simulink library "TM_MASTER"  (Simulink 8.6)
settings: Solver=ode45  StartTime=0.0  StopTime=10.0  RelTol=1e-3
libraries: cdsFilt x75, VIS_LIB x63, cdsEpicsOut x60, cdsTP x48, cdsMuxMatrix x17, cdsFiltCtrl x15, lockin x10, QPD x10, cdsRms x6, FOUROSEM_COILOUTF_MASTER x5, cdsFunctionCall x5, CRYP_TM_MASTER x3
(part 1 of 9)
settings Model: Creator=controls  LastModifiedBy=controls

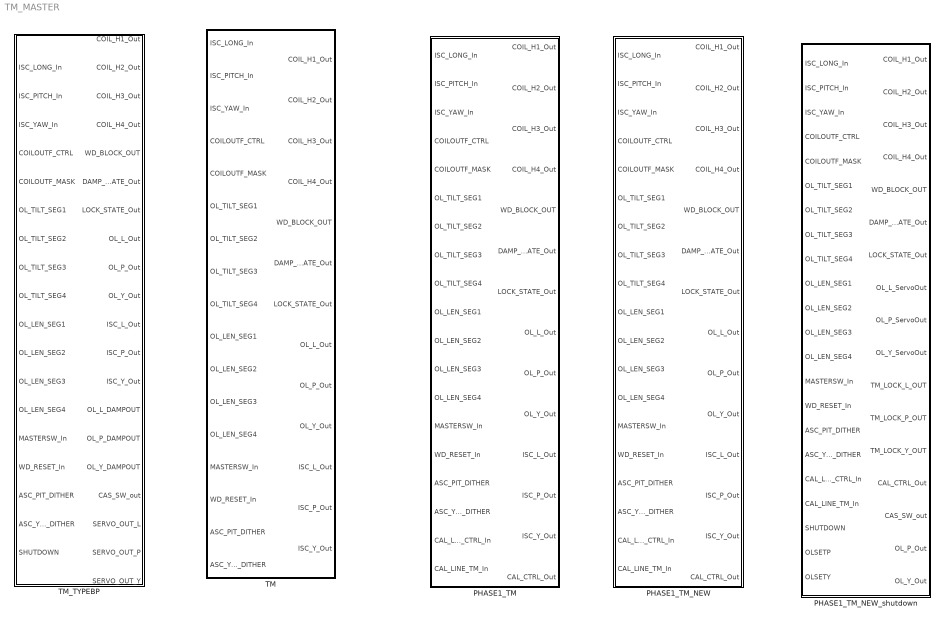
== system TM_MASTER ==
  PHASE1_TM : Subsystem
  PHASE1_TM_NEW : Subsystem
  PHASE1_TM_NEW_shutdown : Subsystem
  TM : Subsystem
  TM_TYPEBP : Subsystem

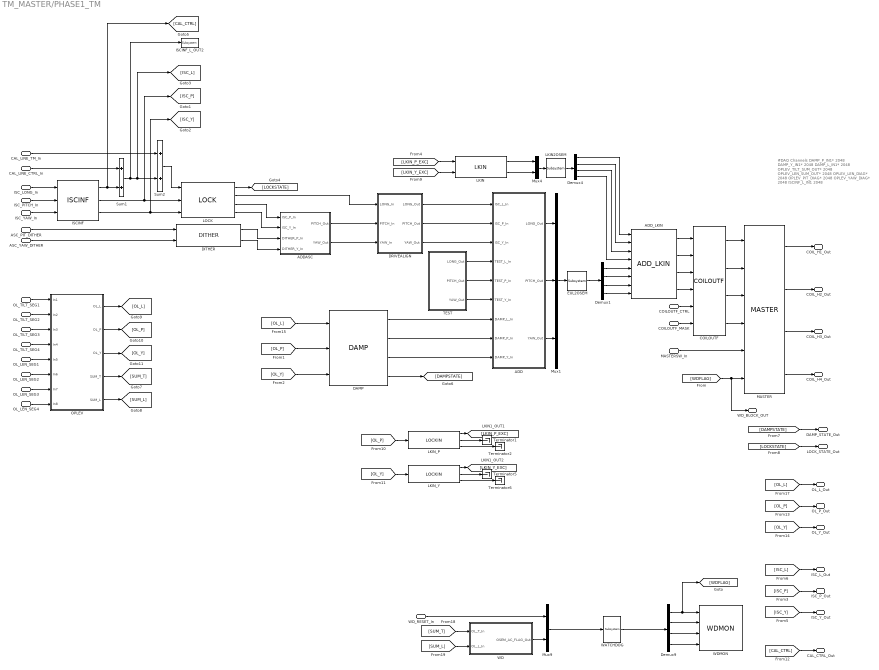
== system TM_MASTER/PHASE1_TM ==
  note: #DAQ Channels
      | DAMP_P_IN1* 2048
      | DAMP_Y_IN1* 2048
      | DAMP_L_IN1* 2048
      | OPLEV_TILT_SUM_OUT* 2048
      | OPLEV_LEN_SUM_OUT* 2048
      | OPLEV_LEN_DIAG* 2048
      | OPLEV_PIT_DIAG* 2048
      | OPLEV_YAW_DIAG* 2048
      | ISCINF_L_IN1 2048
  ISC_LONG_In : Inport
  ISC_PITCH_In : Inport  Port=2
  ISC_YAW_In : Inport  Port=3
  COILOUTF_CTRL : Inport  Port=4
  COILOUTF_MASK : Inport  Port=5
  OL_TILT_SEG1 : Inport  Port=6
  OL_TILT_SEG2 : Inport  Port=7
  OL_TILT_SEG3 : Inport  Port=8
  OL_TILT_SEG4 : Inport  Port=9
  OL_LEN_SEG1 : Inport  Port=10
  OL_LEN_SEG2 : Inport  Port=11
  OL_LEN_SEG3 : Inport  Port=12
  OL_LEN_SEG4 : Inport  Port=13
  MASTERSW_In : Inport  Port=14
  WD_RESET_In : Inport  Port=15
  ASC_PIT_DITHER : Inport  Port=16
  ASC_YAW_DITHER : Inport  Port=17
  CAL_LINE_CTRL_In : Inport  Port=18
  CAL_LINE_TM_In : Inport  Port=19
  ADD : Subsystem
  ADDASC : Subsystem
  ADD_LKIN : VIS_LIB/ADD_LKIN
  COILOUTF : FOUROSEM_COILOUTF_MASTER/COILOUTF
  DAMP : VIS_LIB/DAMP
  DITHER : VIS_LIB/DITHER
  DRIVEALIGN : Subsystem
  Demux1 : Demux
  Demux4 : Demux
  Demux9 : Demux
  EUL2OSEM : cdsMuxMatrix/Subsystem  Tag=cdsMuxMatrix  Description=Any size matrix. Inputs and outputs must be connected using Mux and Demux parts.
      settings: AttributesFormatString=%<Tag>
  ISCINF : VIS_LIB/ISCINF
  ISCINF_L_OUT2 : cdsTP/Subsystem  Tag=Test Point
      settings: AttributesFormatString=%<Tag>
  LKIN : VIS_LIB/LKIN
  LKIN2OSEM : cdsMuxMatrix/Subsystem  Tag=cdsMuxMatrix  Description=Any size matrix. Inputs and outputs must be connected using Mux and Demux parts.
      settings: AttributesFormatString=%<Tag>
  LKIN_P : lockin/LOCKIN  Description=ADL=LOCKIN.adl
      settings: AttributesFormatString=%<Tag>
  LKIN_Y : lockin/LOCKIN  Description=ADL=LOCKIN.adl
      settings: AttributesFormatString=%<Tag>
  LOCK : VIS_LIB/LOCK
  MASTER : CRYP_TM_MASTER/CRYP_TM_MASTER/MASTER
  Mux1 : Mux  Inputs=3
  Mux4 : Mux  Inputs=2
  Mux9 : Mux  Inputs=2
  OPLEV : Subsystem
  Sum1 : Sum
  Sum2 : Sum
  TEST : Subsystem
  Terminator{1..2,5..6} (4 alike) : Terminator
  WATCHDOG : cdsFunctionCall/Subsystem  Tag=cdsFunctionCall  Description=inline OSEMWATCHDOG /opt/rtcds/userapps/release/vis/common/src/WATCHDOG.c
      settings: AttributesFormatString=%<Tag>\n%<Description>
  WD : Subsystem
  WDMON : VIS_LIB/WDMON
  COIL_H1_Out : Outport
  COIL_H2_Out : Outport  Port=2
  COIL_H3_Out : Outport  Port=3
  COIL_H4_Out : Outport  Port=4
  WD_BLOCK_OUT : Outport  Port=5
  DAMP_STATE_Out : Outport  Port=6
  LOCK_STATE_Out : Outport  Port=7
  OL_L_Out : Outport  Port=8
  OL_P_Out : Outport  Port=9
  OL_Y_Out : Outport  Port=10
  ISC_L_Out : Outport  Port=11
  ISC_P_Out : Outport  Port=12
  ISC_Y_Out : Outport  Port=13
  CAL_CTRL_Out : Outport  Port=14
  wires:
  [OL_Y] -> OL_Y_Out/1
  [OL_P] -> OL_P_Out/1
  ISC_PITCH_In/1 -> ISCINF/2
  ISC_LONG_In/1 -> ISCINF/1
  ISC_YAW_In/1 -> ISCINF/3
  WD/1(OSEM_AC_FLAG_Out) -> Mux9/2
  [LKIN_Y_EXC] -> LKIN/2
  [LKIN_P_EXC] -> LKIN/1
  LKIN_Y/3 -> Terminator6/1
  LKIN_Y/2 -> Terminator5/1
  [OL_Y] -> LKIN_Y/1
  LKIN_Y/1 -> [LKIN_Y_EXC]
  LKIN_P/1 -> [LKIN_P_EXC]
  LKIN_P/3 -> Terminator2/1
  LKIN_P/2 -> Terminator1/1
  [OL_P] -> LKIN_P/1
  LOCK/1 -> [LOCKSTATE]
  [LOCKSTATE] -> LOCK_STATE_Out/1
  [DAMPSTATE] -> DAMP_STATE_Out/1
  MASTERSW_In/1 -> MASTER/5
  ADD_LKIN/4 -> COILOUTF/4
  ADD_LKIN/3 -> COILOUTF/3
  ADD_LKIN/2 -> COILOUTF/2
  ADD_LKIN/1 -> COILOUTF/1
  Demux1/4 -> ADD_LKIN/8
  Demux1/3 -> ADD_LKIN/7
  Demux1/2 -> ADD_LKIN/6
  Demux1/1 -> ADD_LKIN/5
  Demux4/4 -> ADD_LKIN/4
  Demux4/3 -> ADD_LKIN/3
  Demux4/2 -> ADD_LKIN/2
  LKIN/2 -> Mux4/2
  LKIN/1 -> Mux4/1
  Demux4/1 -> ADD_LKIN/1
  LKIN2OSEM/1 -> Demux4/1
  Mux4/1 -> LKIN2OSEM/1
  MASTER/4 -> COIL_H4_Out/1
  MASTER/3 -> COIL_H3_Out/1
  MASTER/2 -> COIL_H2_Out/1
  MASTER/1 -> COIL_H1_Out/1
  DRIVEALIGN/3(YAW_Out) -> ADD/3(ISC_Y_In)
  DRIVEALIGN/2(PITCH_Out) -> ADD/2(ISC_P_In)
  DRIVEALIGN/1(LONG_Out) -> ADD/1(ISC_L_In)
  ADDASC/2(YAW_Out) -> DRIVEALIGN/3(YAW_In)
  ADDASC/1(PITCH_Out) -> DRIVEALIGN/2(PITCH_In)
  LOCK/2 -> DRIVEALIGN/1(LONG_In)
  ADD/1(LONG_Out) -> Mux1/1
  ADD/2(PITCH_Out) -> Mux1/2
  ADD/3(YAW_Out) -> Mux1/3
  DITHER/2 -> ADDASC/4(DITHER_Y_In)
  DITHER/1 -> ADDASC/3(DITHER_P_In)
  LOCK/4 -> ADDASC/2(ISC_Y_In)
  ASC_YAW_DITHER/1 -> DITHER/2
  ASC_PIT_DITHER/1 -> DITHER/1
  Mux1/1 -> EUL2OSEM/1
  EUL2OSEM/1 -> Demux1/1
  Demux9/1 -> [WDFLAG], WDMON/1
  Demux9/2 -> WDMON/2
  Demux9/3 -> WDMON/3
  Demux9/4 -> WDMON/4
  WATCHDOG/1 -> Demux9/1
  Mux9/1 -> WATCHDOG/1
  [WDFLAG] -> WD_BLOCK_OUT/1, MASTER/6
  COILOUTF/1 -> MASTER/1
  COILOUTF/2 -> MASTER/2
  COILOUTF/3 -> MASTER/3
  COILOUTF/4 -> MASTER/4
  WD_RESET_In/1 -> Mux9/1
  COILOUTF_MASK/1 -> COILOUTF/6
  COILOUTF_CTRL/1 -> COILOUTF/5
  TEST/1(LONG_Out) -> ADD/4(TEST_L_In)
  TEST/2(PITCH_Out) -> ADD/5(TEST_P_In)
  TEST/3(YAW_Out) -> ADD/6(TEST_Y_In)
  LOCK/3 -> ADDASC/1(ISC_P_In)
  OL_TILT_SEG1/1 -> OPLEV/1(In1)
  OL_TILT_SEG2/1 -> OPLEV/2(In2)
  OL_TILT_SEG4/1 -> OPLEV/4(In4)
  OL_LEN_SEG1/1 -> OPLEV/5(In5)
  OL_LEN_SEG2/1 -> OPLEV/6(In6)
  OL_LEN_SEG3/1 -> OPLEV/7(In7)
  OL_LEN_SEG4/1 -> OPLEV/8(In8)
  OL_TILT_SEG3/1 -> OPLEV/3(In3)
  [OL_L] -> DAMP/1
  DAMP/4 -> [DAMPSTATE]
  DAMP/1 -> ADD/7(DAMP_L_In)
  [SUM_T] -> WD/1(OL_T_In)
  OPLEV/4(SUM_T) -> [SUM_T]
  OPLEV/5(SUM_L) -> [SUM_L]
  [SUM_L] -> WD/2(OL_L_In)
  [OL_L] -> OL_L_Out/1
  OPLEV/1(OL_L) -> [OL_L]
  OPLEV/2(OL_P) -> [OL_P]
  OPLEV/3(OL_Y) -> [OL_Y]
  DAMP/2 -> ADD/8(DAMP_P_In)
  DAMP/3 -> ADD/9(DAMP_Y_In)
  [OL_P] -> DAMP/2
  [OL_Y] -> DAMP/3
  ISCINF/2 -> LOCK/2, [ISC_P]
  ISCINF/3 -> LOCK/3, [ISC_Y]
  [ISC_Y] -> ISC_Y_Out/1
  [ISC_P] -> ISC_P_Out/1
  [ISC_L] -> ISC_L_Out/1
  ISCINF/1 -> [CAL_CTRL], Sum1/2
  CAL_LINE_CTRL_In/1 -> Sum1/1
  Sum1/1 -> ISCINF_L_OUT2/1, [ISC_L], Sum2/2
  CAL_LINE_TM_In/1 -> Sum2/1
  Sum2/1 -> LOCK/1
  [CAL_CTRL] -> CAL_CTRL_Out/1

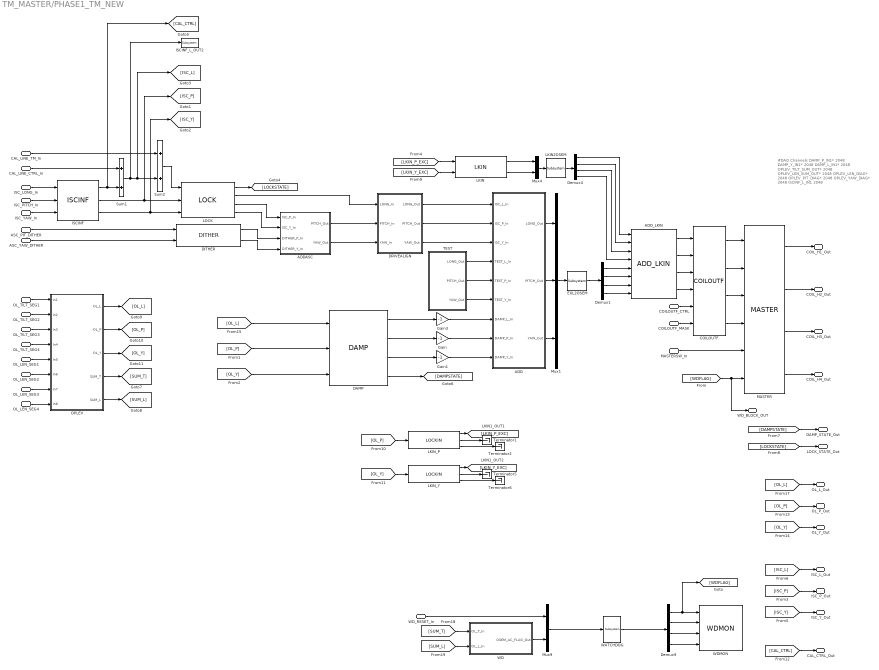
== system TM_MASTER/PHASE1_TM_NEW ==
  note: #DAQ Channels
      | DAMP_P_IN1* 2048
      | DAMP_Y_IN1* 2048
      | DAMP_L_IN1* 2048
      | OPLEV_TILT_SUM_OUT* 2048
      | OPLEV_LEN_SUM_OUT* 2048
      | OPLEV_LEN_DIAG* 2048
      | OPLEV_PIT_DIAG* 2048
      | OPLEV_YAW_DIAG* 2048
      | ISCINF_L_IN1 2048
  ISC_LONG_In : Inport
  ISC_PITCH_In : Inport  Port=2
  ISC_YAW_In : Inport  Port=3
  COILOUTF_CTRL : Inport  Port=4
  COILOUTF_MASK : Inport  Port=5
  OL_TILT_SEG1 : Inport  Port=6
  OL_TILT_SEG2 : Inport  Port=7
  OL_TILT_SEG3 : Inport  Port=8
  OL_TILT_SEG4 : Inport  Port=9
  OL_LEN_SEG1 : Inport  Port=10
  OL_LEN_SEG2 : Inport  Port=11
  OL_LEN_SEG3 : Inport  Port=12
  OL_LEN_SEG4 : Inport  Port=13
  MASTERSW_In : Inport  Port=14
  WD_RESET_In : Inport  Port=15
  ASC_PIT_DITHER : Inport  Port=16
  ASC_YAW_DITHER : Inport  Port=17
  CAL_LINE_CTRL_In : Inport  Port=18
  CAL_LINE_TM_In : Inport  Port=19
  ADD : Subsystem
  ADDASC : Subsystem
  ADD_LKIN : VIS_LIB/ADD_LKIN
  COILOUTF : FOUROSEM_COILOUTF_MASTER/COILOUTF
  DAMP : VIS_LIB/DAMP
  DITHER : VIS_LIB/DITHER
  DRIVEALIGN : Subsystem
  Demux1 : Demux
  Demux4 : Demux
  Demux9 : Demux
  EUL2OSEM : cdsMuxMatrix/Subsystem  Tag=cdsMuxMatrix  Description=Any size matrix. Inputs and outputs must be connected using Mux and Demux parts.
      settings: AttributesFormatString=%<Tag>
  Gain : Gain  Gain=-1
  Gain1 : Gain  Gain=-1
  Gain3 : Gain  Gain=-1
  ISCINF : VIS_LIB/ISCINF
  ISCINF_L_OUT2 : cdsTP/Subsystem  Tag=Test Point
      settings: AttributesFormatString=%<Tag>
  LKIN : VIS_LIB/LKIN
  LKIN2OSEM : cdsMuxMatrix/Subsystem  Tag=cdsMuxMatrix  Description=Any size matrix. Inputs and outputs must be connected using Mux and Demux parts.
      settings: AttributesFormatString=%<Tag>
  LKIN_P : lockin/LOCKIN  Description=ADL=LOCKIN.adl
      settings: AttributesFormatString=%<Tag>
  LKIN_Y : lockin/LOCKIN  Description=ADL=LOCKIN.adl
      settings: AttributesFormatString=%<Tag>
  LOCK : VIS_LIB/LOCK
  MASTER : CRYP_TM_MASTER/CRYP_TM_MASTER/MASTER
  Mux1 : Mux  Inputs=3
  Mux4 : Mux  Inputs=2
  Mux9 : Mux  Inputs=2
  OPLEV : Subsystem
  Sum1 : Sum
  Sum2 : Sum
  TEST : Subsystem
  Terminator{1..2,5..6} (4 alike) : Terminator
  WATCHDOG : cdsFunctionCall/Subsystem  Tag=cdsFunctionCall  Description=inline OSEMWATCHDOG /opt/rtcds/userapps/release/vis/common/src/WATCHDOG.c
      settings: AttributesFormatString=%<Tag>\n%<Description>
  WD : Subsystem
  WDMON : VIS_LIB/WDMON
  COIL_H1_Out : Outport
  COIL_H2_Out : Outport  Port=2
  COIL_H3_Out : Outport  Port=3
  COIL_H4_Out : Outport  Port=4
  WD_BLOCK_OUT : Outport  Port=5
  DAMP_STATE_Out : Outport  Port=6
  LOCK_STATE_Out : Outport  Port=7
  OL_L_Out : Outport  Port=8
  OL_P_Out : Outport  Port=9
  OL_Y_Out : Outport  Port=10
  ISC_L_Out : Outport  Port=11
  ISC_P_Out : Outport  Port=12
  ISC_Y_Out : Outport  Port=13
  CAL_CTRL_Out : Outport  Port=14
  wires:
  [OL_Y] -> OL_Y_Out/1
  [OL_P] -> OL_P_Out/1
  ISC_PITCH_In/1 -> ISCINF/2
  ISC_LONG_In/1 -> ISCINF/1
  ISC_YAW_In/1 -> ISCINF/3
  WD/1(OSEM_AC_FLAG_Out) -> Mux9/2
  [LKIN_Y_EXC] -> LKIN/2
  [LKIN_P_EXC] -> LKIN/1
  LKIN_Y/3 -> Terminator6/1
  LKIN_Y/2 -> Terminator5/1
  [OL_Y] -> LKIN_Y/1
  LKIN_Y/1 -> [LKIN_Y_EXC]
  LKIN_P/1 -> [LKIN_P_EXC]
  LKIN_P/3 -> Terminator2/1
  LKIN_P/2 -> Terminator1/1
  [OL_P] -> LKIN_P/1
  LOCK/1 -> [LOCKSTATE]
  [LOCKSTATE] -> LOCK_STATE_Out/1
  [DAMPSTATE] -> DAMP_STATE_Out/1
  MASTERSW_In/1 -> MASTER/5
  ADD_LKIN/4 -> COILOUTF/4
  ADD_LKIN/3 -> COILOUTF/3
  ADD_LKIN/2 -> COILOUTF/2
  ADD_LKIN/1 -> COILOUTF/1
  Demux1/4 -> ADD_LKIN/8
  Demux1/3 -> ADD_LKIN/7
  Demux1/2 -> ADD_LKIN/6
  Demux1/1 -> ADD_LKIN/5
  Demux4/4 -> ADD_LKIN/4
  Demux4/3 -> ADD_LKIN/3
  Demux4/2 -> ADD_LKIN/2
  LKIN/2 -> Mux4/2
  LKIN/1 -> Mux4/1
  Demux4/1 -> ADD_LKIN/1
  LKIN2OSEM/1 -> Demux4/1
  Mux4/1 -> LKIN2OSEM/1
  MASTER/4 -> COIL_H4_Out/1
  MASTER/3 -> COIL_H3_Out/1
  MASTER/2 -> COIL_H2_Out/1
  MASTER/1 -> COIL_H1_Out/1
  DRIVEALIGN/3(YAW_Out) -> ADD/3(ISC_Y_In)
  DRIVEALIGN/2(PITCH_Out) -> ADD/2(ISC_P_In)
  DRIVEALIGN/1(LONG_Out) -> ADD/1(ISC_L_In)
  ADDASC/2(YAW_Out) -> DRIVEALIGN/3(YAW_In)
  ADDASC/1(PITCH_Out) -> DRIVEALIGN/2(PITCH_In)
  LOCK/2 -> DRIVEALIGN/1(LONG_In)
  ADD/1(LONG_Out) -> Mux1/1
  ADD/2(PITCH_Out) -> Mux1/2
  ADD/3(YAW_Out) -> Mux1/3
  DITHER/2 -> ADDASC/4(DITHER_Y_In)
  DITHER/1 -> ADDASC/3(DITHER_P_In)
  LOCK/4 -> ADDASC/2(ISC_Y_In)
  ASC_YAW_DITHER/1 -> DITHER/2
  ASC_PIT_DITHER/1 -> DITHER/1
  Mux1/1 -> EUL2OSEM/1
  EUL2OSEM/1 -> Demux1/1
  Demux9/1 -> [WDFLAG], WDMON/1
  Demux9/2 -> WDMON/2
  Demux9/3 -> WDMON/3
  Demux9/4 -> WDMON/4
  WATCHDOG/1 -> Demux9/1
  Mux9/1 -> WATCHDOG/1
  [WDFLAG] -> WD_BLOCK_OUT/1, MASTER/6
  COILOUTF/1 -> MASTER/1
  COILOUTF/2 -> MASTER/2
  COILOUTF/3 -> MASTER/3
  COILOUTF/4 -> MASTER/4
  WD_RESET_In/1 -> Mux9/1
  COILOUTF_MASK/1 -> COILOUTF/6
  COILOUTF_CTRL/1 -> COILOUTF/5
  TEST/1(LONG_Out) -> ADD/4(TEST_L_In)
  TEST/2(PITCH_Out) -> ADD/5(TEST_P_In)
  TEST/3(YAW_Out) -> ADD/6(TEST_Y_In)
  LOCK/3 -> ADDASC/1(ISC_P_In)
  OL_TILT_SEG1/1 -> OPLEV/1(In1)
  OL_TILT_SEG2/1 -> OPLEV/2(In2)
  OL_TILT_SEG4/1 -> OPLEV/4(In4)
  OL_LEN_SEG1/1 -> OPLEV/5(In5)
  OL_LEN_SEG2/1 -> OPLEV/6(In6)
  OL_LEN_SEG3/1 -> OPLEV/7(In7)
  OL_LEN_SEG4/1 -> OPLEV/8(In8)
  OL_TILT_SEG3/1 -> OPLEV/3(In3)
  DAMP/4 -> [DAMPSTATE]
  DAMP/1 -> Gain3/1
  [SUM_T] -> WD/1(OL_T_In)
  OPLEV/4(SUM_T) -> [SUM_T]
  OPLEV/5(SUM_L) -> [SUM_L]
  [SUM_L] -> WD/2(OL_L_In)
  [OL_L] -> OL_L_Out/1
  OPLEV/1(OL_L) -> [OL_L]
  OPLEV/2(OL_P) -> [OL_P]
  OPLEV/3(OL_Y) -> [OL_Y]
  DAMP/2 -> Gain/1
  DAMP/3 -> Gain1/1
  ISCINF/2 -> LOCK/2, [ISC_P]
  ISCINF/3 -> LOCK/3, [ISC_Y]
  [ISC_Y] -> ISC_Y_Out/1
  [ISC_P] -> ISC_P_Out/1
  [ISC_L] -> ISC_L_Out/1
  ISCINF/1 -> [CAL_CTRL], Sum1/2
  CAL_LINE_CTRL_In/1 -> Sum1/1
  Sum1/1 -> ISCINF_L_OUT2/1, [ISC_L], Sum2/2
  CAL_LINE_TM_In/1 -> Sum2/1
  Sum2/1 -> LOCK/1
  [CAL_CTRL] -> CAL_CTRL_Out/1
  [OL_L] -> DAMP/1
  [OL_P] -> DAMP/2
  [OL_Y] -> DAMP/3
  Gain3/1 -> ADD/7(DAMP_L_In)
  Gain/1 -> ADD/8(DAMP_P_In)
  Gain1/1 -> ADD/9(DAMP_Y_In)

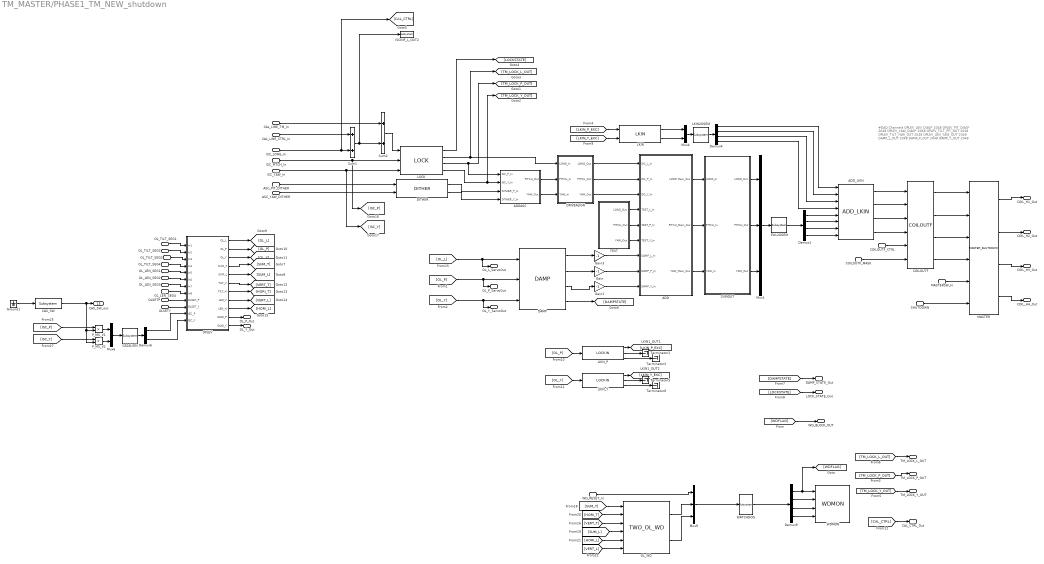
== system TM_MASTER/PHASE1_TM_NEW_shutdown ==
  note: #DAQ Channels
      | OPLEV_LEN_DIAG* 2048
      | OPLEV_PIT_DIAG* 2048
      | OPLEV_YAW_DIAG* 2048
      | OPLEV_TILT_PIT_OUT 2048
      | OPLEV_TILT_YAW_OUT 2048
      | OPLEV_LEN_YAW_OUT 2048
      | DAMP_L_OUT 2048
      | DAMP_P_OUT 2048
      | DAMP_Y_OUT 2048
  ISC_LONG_In : Inport
  ISC_PITCH_In : Inport  Port=2
  ISC_YAW_In : Inport  Port=3
  COILOUTF_CTRL : Inport  Port=4
  COILOUTF_MASK : Inport  Port=5
  OL_TILT_SEG1 : Inport  Port=6
  OL_TILT_SEG2 : Inport  Port=7
  OL_TILT_SEG3 : Inport  Port=8
  OL_TILT_SEG4 : Inport  Port=9
  OL_LEN_SEG1 : Inport  Port=10
  OL_LEN_SEG2 : Inport  Port=11
  OL_LEN_SEG3 : Inport  Port=12
  OL_LEN_SEG4 : Inport  Port=13
  MASTERSW_In : Inport  Port=14
  WD_RESET_In : Inport  Port=15
  ASC_PIT_DITHER : Inport  Port=16
  ASC_YAW_DITHER : Inport  Port=17
  CAL_LINE_CTRL_In : Inport  Port=18
  CAL_LINE_TM_In : Inport  Port=19
  SHUTDOWN : Inport  Port=20
  OLSETP : Inport  Port=21
  OLSETY : Inport  Port=22
  ADD : Subsystem
  ADDASC : Subsystem
  ADD_LKIN : VIS_LIB/ADD_LKIN
  CASALIGN : cdsMuxMatrix/Subsystem  Tag=cdsMuxMatrix  Description=Any size matrix. Inputs and outputs must be connected using Mux and Demux parts.
      settings: AttributesFormatString=%<Tag>
  CAS_SW : cdsEpicsBinIn/Subsystem  Tag=cdsEpicsBinIn  Description=|
      | Purpose:                                                                            
      | Create an EPICS binary (0 or 1) input channel to the FE realtime controls.          
      |                                                                                     
      | Operation:                                                                          
      | Outputs value from an EPICS ai record. Value is binary input (bi Epics record type).
      |                                                                                     
      | Usage:                                                                              
      | Name the part with the desired EPICS channel name.
      settings: AttributesFormatString=%<Tag>
  COILOUTF : FOUROSEM_COILOUTF_MASTER/COILOUTF
  DAMP : VIS_LIB/DAMP
  DITHER : VIS_LIB/DITHER
  DRIVEALIGN : Subsystem
  Demux1 : Demux
  Demux4 : Demux
  Demux6 : Demux  Outputs=2
  Demux9 : Demux
  EUL2OSEM : cdsMuxMatrix/Subsystem  Tag=cdsMuxMatrix  Description=Any size matrix. Inputs and outputs must be connected using Mux and Demux parts.
      settings: AttributesFormatString=%<Tag>
  Gain : Gain  Gain=-1
  Gain1 : Gain  Gain=-1
  Gain3 : Gain  Gain=-1
  Ground1 : Ground
  ISCINF_L_OUT2 : cdsTP/Subsystem  Tag=Test Point
      settings: AttributesFormatString=%<Tag>
  LKIN : VIS_LIB/LKIN
  LKIN2OSEM : cdsMuxMatrix/Subsystem  Tag=cdsMuxMatrix  Description=Any size matrix. Inputs and outputs must be connected using Mux and Demux parts.
      settings: AttributesFormatString=%<Tag>
  LKIN_P : lockin/LOCKIN  Description=ADL=LOCKIN.adl
      settings: AttributesFormatString=%<Tag>
  LKIN_Y : lockin/LOCKIN  Description=ADL=LOCKIN.adl
      settings: AttributesFormatString=%<Tag>
  LOCK : VIS_LIB/LOCK
  MASTER : VIS_LIB/MASTER_SHUTDOWN
  Mux1 : Mux  Inputs=3
  Mux4 : Mux  Inputs=2
  Mux6 : Mux  Inputs=2
  Mux9 : Mux  Inputs=3
  OL_WD : OPLEV_MASTER/TWO_OL_WD
  OPLEV : Subsystem
  P_MS_V1 : Product  RndMeth=Zero
  P_MS_V2 : Product  RndMeth=Zero
  SUMOUT : Subsystem
  Sum1 : Sum
  Sum2 : Sum
  TEST : Subsystem
  Terminator{1..2,5..6} (4 alike) : Terminator
  WATCHDOG : cdsFunctionCall/Subsystem  Tag=cdsFunctionCall  Description=inline OPLEVWATCHDOG /opt/rtcds/userapps/release/vis/common/src/WATCHDOG.c
      settings: AttributesFormatString=%<Tag>\n%<Description>
  WDMON : VIS_LIB/WDMON
  COIL_H1_Out : Outport
  COIL_H2_Out : Outport  Port=2
  COIL_H3_Out : Outport  Port=3
  COIL_H4_Out : Outport  Port=4
  WD_BLOCK_OUT : Outport  Port=5
  DAMP_STATE_Out : Outport  Port=6
  LOCK_STATE_Out : Outport  Port=7
  OL_L_ServoOut : Outport  Port=8
  OL_P_ServoOut : Outport  Port=9
  OL_Y_ServoOut : Outport  Port=10
  TM_LOCK_L_OUT : Outport  Port=11
  TM_LOCK_P_OUT : Outport  Port=12
  TM_LOCK_Y_OUT : Outport  Port=13
  CAL_CTRL_Out : Outport  Port=14
  CAS_SW_out : Outport  Port=15
  OL_P_Out : Outport  Port=16
  OL_Y_Out : Outport  Port=17
  wires:
  CASALIGN/1 -> Demux6/1
  Mux6/1 -> CASALIGN/1
  P_MS_V2/1 -> Mux6/2
  P_MS_V1/1 -> Mux6/1
  CAS_SW/1 -> CAS_SW_out/1, P_MS_V2/2, P_MS_V1/2
  [ISC_P] -> P_MS_V1/1
  [ISC_Y] -> P_MS_V2/1
  Ground1/1 -> CAS_SW/1
  OPLEV/3(OL_Y) -> [OL_Y]
  SUMOUT/3(YAW_Out) -> Mux1/3
  SUMOUT/2(PITCH_Out) -> Mux1/2
  SUMOUT/1(LONG_Out) -> Mux1/1
  OL_WD/1 -> Mux9/2
  [LKIN_Y_EXC] -> LKIN/2
  [LKIN_P_EXC] -> LKIN/1
  LKIN_Y/3 -> Terminator6/1
  LKIN_Y/2 -> Terminator5/1
  [OL_Y] -> LKIN_Y/1
  LKIN_Y/1 -> [LKIN_Y_EXC]
  LKIN_P/1 -> [LKIN_P_EXC]
  LKIN_P/3 -> Terminator2/1
  LKIN_P/2 -> Terminator1/1
  [OL_P] -> LKIN_P/1
  LOCK/1 -> [LOCKSTATE]
  [LOCKSTATE] -> LOCK_STATE_Out/1
  [DAMPSTATE] -> DAMP_STATE_Out/1
  MASTERSW_In/1 -> MASTER/5
  ADD_LKIN/4 -> COILOUTF/4
  ADD_LKIN/3 -> COILOUTF/3
  ADD_LKIN/2 -> COILOUTF/2
  ADD_LKIN/1 -> COILOUTF/1
  Demux1/4 -> ADD_LKIN/8
  Demux1/3 -> ADD_LKIN/7
  Demux1/2 -> ADD_LKIN/6
  Demux1/1 -> ADD_LKIN/5
  Demux4/4 -> ADD_LKIN/4
  Demux4/3 -> ADD_LKIN/3
  Demux4/2 -> ADD_LKIN/2
  LKIN/2 -> Mux4/2
  LKIN/1 -> Mux4/1
  Demux4/1 -> ADD_LKIN/1
  LKIN2OSEM/1 -> Demux4/1
  Mux4/1 -> LKIN2OSEM/1
  MASTER/4 -> COIL_H4_Out/1
  MASTER/3 -> COIL_H3_Out/1
  MASTER/2 -> COIL_H2_Out/1
  MASTER/1 -> COIL_H1_Out/1
  DRIVEALIGN/3(YAW_Out) -> ADD/3(ISC_Y_In)
  DRIVEALIGN/2(PITCH_Out) -> ADD/2(ISC_P_In)
  DRIVEALIGN/1(LONG_Out) -> ADD/1(ISC_L_In)
  ADDASC/2(YAW_Out) -> DRIVEALIGN/3(YAW_In)
  ADDASC/1(PITCH_Out) -> DRIVEALIGN/2(PITCH_In)
  LOCK/2 -> [TM_LOCK_L_OUT], DRIVEALIGN/1(LONG_In)
  ADD/1(LONG Main_Out) -> SUMOUT/1(LONG_In)
  ADD/2(PITCH_Main_Out) -> SUMOUT/2(PITCH_In)
  ADD/3(YAW_Main_Out) -> SUMOUT/3(YAW_In)
  DITHER/2 -> ADDASC/4(DITHER_Y_In)
  DITHER/1 -> ADDASC/3(DITHER_P_In)
  LOCK/4 -> [TM_LOCK_Y_OUT], ADDASC/2(ISC_Y_In)
  ASC_YAW_DITHER/1 -> DITHER/2
  ASC_PIT_DITHER/1 -> DITHER/1
  Mux1/1 -> EUL2OSEM/1
  EUL2OSEM/1 -> Demux1/1
  Demux9/1 -> [WDFLAG], WDMON/1
  Demux9/2 -> WDMON/2
  Demux9/3 -> WDMON/3
  Demux9/4 -> WDMON/4
  WATCHDOG/1 -> Demux9/1
  Mux9/1 -> WATCHDOG/1
  [WDFLAG] -> WD_BLOCK_OUT/1
  COILOUTF/1 -> MASTER/1
  COILOUTF/2 -> MASTER/2
  COILOUTF/3 -> MASTER/3
  COILOUTF/4 -> MASTER/4
  WD_RESET_In/1 -> Mux9/1
  COILOUTF_MASK/1 -> COILOUTF/6
  COILOUTF_CTRL/1 -> COILOUTF/5
  TEST/1(LONG_Out) -> ADD/4(TEST_L_In)
  TEST/2(PITCH_Out) -> ADD/5(TEST_P_In)
  TEST/3(YAW_Out) -> ADD/6(TEST_Y_In)
  LOCK/3 -> [TM_LOCK_P_OUT], ADDASC/1(ISC_P_In)
  OL_TILT_SEG1/1 -> OPLEV/1(In1)
  OL_TILT_SEG2/1 -> OPLEV/2(In2)
  OL_TILT_SEG4/1 -> OPLEV/4(In4)
  OL_LEN_SEG1/1 -> OPLEV/5(In5)
  OL_LEN_SEG2/1 -> OPLEV/6(In6)
  OL_LEN_SEG3/1 -> OPLEV/7(In7)
  OL_LEN_SEG4/1 -> OPLEV/8(In8)
  OL_TILT_SEG3/1 -> OPLEV/3(In3)
  DAMP/4 -> [DAMPSTATE]
  DAMP/1 -> Gain3/1
  [SUM_T] -> OL_WD/1
  OPLEV/4(SUM_T) -> [SUM_T]
  OPLEV/5(SUM_L) -> [SUM_L]
  [SUM_L] -> OL_WD/4
  OPLEV/1(OL_L) -> [OL_L]
  DAMP/2 -> Gain/1
  DAMP/3 -> Gain1/1
  ISC_PITCH_In/1 -> LOCK/2, [ISC_P]
  ISC_YAW_In/1 -> LOCK/3, [ISC_Y]
  [TM_LOCK_Y_OUT] -> TM_LOCK_Y_OUT/1
  [TM_LOCK_P_OUT] -> TM_LOCK_P_OUT/1
  [TM_LOCK_L_OUT] -> TM_LOCK_L_OUT/1
  ISC_LONG_In/1 -> [CAL_CTRL], Sum1/2
  CAL_LINE_CTRL_In/1 -> Sum1/1
  Sum1/1 -> ISCINF_L_OUT2/1, Sum2/2
  CAL_LINE_TM_In/1 -> Sum2/1
  Sum2/1 -> LOCK/1
  [CAL_CTRL] -> CAL_CTRL_Out/1
  [OL_L] -> OL_L_ServoOut/1, DAMP/1
  SHUTDOWN/1 -> MASTER/6
  OPLEV/6(TILT_V) -> [VERT_T]
  OPLEV/7(TILT_H) -> [HORI_T]
  OPLEV/8(LEN_V) -> [VERT_L]
  OPLEV/9(LEN_H) -> [HORI_L]
  OL_WD/2 -> Mux9/3
  [VERT_T] -> OL_WD/3
  [HORI_T] -> OL_WD/2
  [HORI_L] -> OL_WD/5
  [VERT_L] -> OL_WD/6
  OPLEV/2(OL_P) -> [OL_P]
  Demux6/1 -> OPLEV/11(ISC_P)
  Demux6/2 -> OPLEV/12(ISC_Y)
  Gain3/1 -> ADD/7(DAMP_L_In)
  Gain/1 -> ADD/8(DAMP_P_In)
  Gain1/1 -> ADD/9(DAMP_Y_In)
  [OL_P] -> OL_P_ServoOut/1, DAMP/2
  [OL_Y] -> OL_Y_ServoOut/1, DAMP/3
  OLSETP/1 -> OPLEV/9(OLSET_P)
  OLSETY/1 -> OPLEV/10(OLSET_Y)
  OPLEV/10(DIAG_P) -> OL_P_Out/1
  OPLEV/11(DIAG_Y) -> OL_Y_Out/1

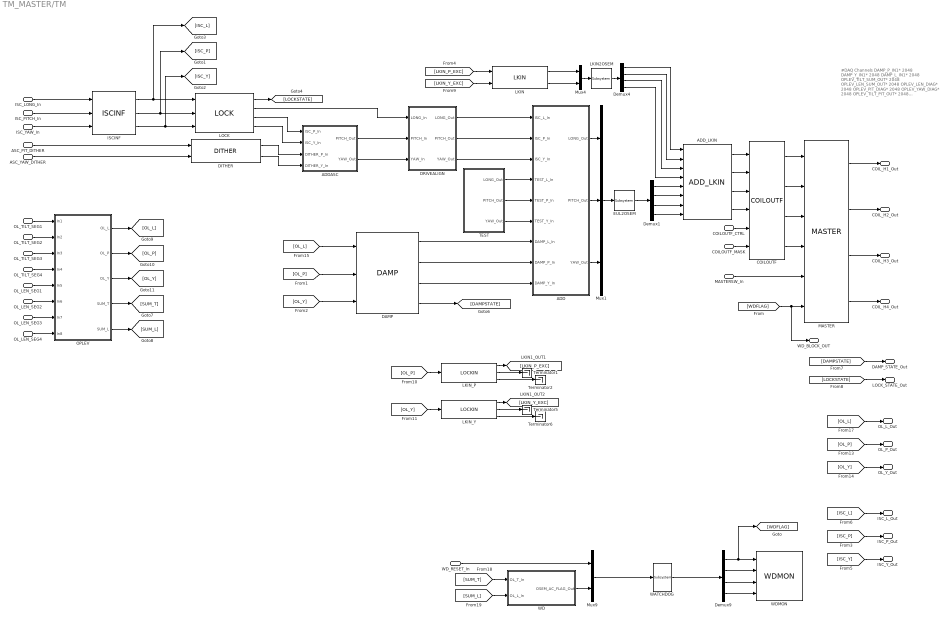
== system TM_MASTER/TM ==
  note: #DAQ Channels
      | DAMP_P_IN1* 2048
      | DAMP_Y_IN1* 2048
      | DAMP_L_IN1* 2048
      | OPLEV_TILT_SUM_OUT* 2048
      | OPLEV_LEN_SUM_OUT* 2048
      | OPLEV_LEN_DIAG* 2048
      | OPLEV_PIT_DIAG* 2048
      | OPLEV_YAW_DIAG* 2048
      | OPLEV_TILT_PIT_OUT* 2048
      | OPLEV_TILT_YAW_OUT* 2048
      | ISCINF_L_IN1 2048
  ISC_LONG_In : Inport
  ISC_PITCH_In : Inport  Port=2
  ISC_YAW_In : Inport  Port=3
  COILOUTF_CTRL : Inport  Port=4
  COILOUTF_MASK : Inport  Port=5
  OL_TILT_SEG1 : Inport  Port=6
  OL_TILT_SEG2 : Inport  Port=7
  OL_TILT_SEG3 : Inport  Port=8
  OL_TILT_SEG4 : Inport  Port=9
  OL_LEN_SEG1 : Inport  Port=10
  OL_LEN_SEG2 : Inport  Port=11
  OL_LEN_SEG3 : Inport  Port=12
  OL_LEN_SEG4 : Inport  Port=13
  MASTERSW_In : Inport  Port=14
  WD_RESET_In : Inport  Port=15
  ASC_PIT_DITHER : Inport  Port=16
  ASC_YAW_DITHER : Inport  Port=17
  ADD : Subsystem
  ADDASC : Subsystem
  ADD_LKIN : VIS_LIB/ADD_LKIN
  COILOUTF : FOUROSEM_COILOUTF_MASTER/COILOUTF
  DAMP : VIS_LIB/DAMP
  DITHER : VIS_LIB/DITHER
  DRIVEALIGN : Subsystem
  Demux1 : Demux
  Demux4 : Demux
  Demux9 : Demux
  EUL2OSEM : cdsMuxMatrix/Subsystem  Tag=cdsMuxMatrix  Description=Any size matrix. Inputs and outputs must be connected using Mux and Demux parts.
      settings: AttributesFormatString=%<Tag>
  ISCINF : VIS_LIB/ISCINF
  LKIN : VIS_LIB/LKIN
  LKIN2OSEM : cdsMuxMatrix/Subsystem  Tag=cdsMuxMatrix  Description=Any size matrix. Inputs and outputs must be connected using Mux and Demux parts.
      settings: AttributesFormatString=%<Tag>
  LKIN_P : lockin/LOCKIN  Description=ADL=LOCKIN.adl
      settings: AttributesFormatString=%<Tag>
  LKIN_Y : lockin/LOCKIN  Description=ADL=LOCKIN.adl
      settings: AttributesFormatString=%<Tag>
  LOCK : VIS_LIB/LOCK
  MASTER : CRYP_TM_MASTER/CRYP_TM_MASTER/MASTER
  Mux1 : Mux  Inputs=3
  Mux4 : Mux  Inputs=2
  Mux9 : Mux  Inputs=2
  OPLEV : Subsystem
  TEST : Subsystem
  Terminator{1..2,5..6} (4 alike) : Terminator
  WATCHDOG : cdsFunctionCall/Subsystem  Tag=cdsFunctionCall  Description=inline OSEMWATCHDOG /opt/rtcds/userapps/release/vis/common/src/WATCHDOG.c
      settings: AttributesFormatString=%<Tag>\n%<Description>
  WD : Subsystem
  WDMON : VIS_LIB/WDMON
  COIL_H1_Out : Outport
  COIL_H2_Out : Outport  Port=2
  COIL_H3_Out : Outport  Port=3
  COIL_H4_Out : Outport  Port=4
  WD_BLOCK_OUT : Outport  Port=5
  DAMP_STATE_Out : Outport  Port=6
  LOCK_STATE_Out : Outport  Port=7
  OL_L_Out : Outport  Port=8
  OL_P_Out : Outport  Port=9
  OL_Y_Out : Outport  Port=10
  ISC_L_Out : Outport  Port=11
  ISC_P_Out : Outport  Port=12
  ISC_Y_Out : Outport  Port=13
  wires:
  [OL_Y] -> OL_Y_Out/1
  [OL_P] -> OL_P_Out/1
  ISC_PITCH_In/1 -> ISCINF/2
  ISC_LONG_In/1 -> ISCINF/1
  ISC_YAW_In/1 -> ISCINF/3
  WD/1(OSEM_AC_FLAG_Out) -> Mux9/2
  [LKIN_Y_EXC] -> LKIN/2
  [LKIN_P_EXC] -> LKIN/1
  LKIN_Y/3 -> Terminator6/1
  LKIN_Y/2 -> Terminator5/1
  [OL_Y] -> LKIN_Y/1
  LKIN_Y/1 -> [LKIN_Y_EXC]
  LKIN_P/1 -> [LKIN_P_EXC]
  LKIN_P/3 -> Terminator2/1
  LKIN_P/2 -> Terminator1/1
  [OL_P] -> LKIN_P/1
  LOCK/1 -> [LOCKSTATE]
  [LOCKSTATE] -> LOCK_STATE_Out/1
  [DAMPSTATE] -> DAMP_STATE_Out/1
  MASTERSW_In/1 -> MASTER/5
  ADD_LKIN/4 -> COILOUTF/4
  ADD_LKIN/3 -> COILOUTF/3
  ADD_LKIN/2 -> COILOUTF/2
  ADD_LKIN/1 -> COILOUTF/1
  Demux1/4 -> ADD_LKIN/8
  Demux1/3 -> ADD_LKIN/7
  Demux1/2 -> ADD_LKIN/6
  Demux1/1 -> ADD_LKIN/5
  Demux4/4 -> ADD_LKIN/4
  Demux4/3 -> ADD_LKIN/3
  Demux4/2 -> ADD_LKIN/2
  LKIN/2 -> Mux4/2
  LKIN/1 -> Mux4/1
  Demux4/1 -> ADD_LKIN/1
  LKIN2OSEM/1 -> Demux4/1
  Mux4/1 -> LKIN2OSEM/1
  MASTER/4 -> COIL_H4_Out/1
  MASTER/3 -> COIL_H3_Out/1
  MASTER/2 -> COIL_H2_Out/1
  MASTER/1 -> COIL_H1_Out/1
  DRIVEALIGN/3(YAW_Out) -> ADD/3(ISC_Y_In)
  DRIVEALIGN/2(PITCH_Out) -> ADD/2(ISC_P_In)
  DRIVEALIGN/1(LONG_Out) -> ADD/1(ISC_L_In)
  ADDASC/2(YAW_Out) -> DRIVEALIGN/3(YAW_In)
  ADDASC/1(PITCH_Out) -> DRIVEALIGN/2(PITCH_In)
  LOCK/2 -> DRIVEALIGN/1(LONG_In)
  ADD/1(LONG_Out) -> Mux1/1
  ADD/2(PITCH_Out) -> Mux1/2
  ADD/3(YAW_Out) -> Mux1/3
  DITHER/2 -> ADDASC/4(DITHER_Y_In)
  DITHER/1 -> ADDASC/3(DITHER_P_In)
  LOCK/4 -> ADDASC/2(ISC_Y_In)
  ASC_YAW_DITHER/1 -> DITHER/2
  ASC_PIT_DITHER/1 -> DITHER/1
  Mux1/1 -> EUL2OSEM/1
  EUL2OSEM/1 -> Demux1/1
  Demux9/1 -> [WDFLAG], WDMON/1
  Demux9/2 -> WDMON/2
  Demux9/3 -> WDMON/3
  Demux9/4 -> WDMON/4
  WATCHDOG/1 -> Demux9/1
  Mux9/1 -> WATCHDOG/1
  [WDFLAG] -> WD_BLOCK_OUT/1, MASTER/6
  COILOUTF/1 -> MASTER/1
  COILOUTF/2 -> MASTER/2
  COILOUTF/3 -> MASTER/3
  COILOUTF/4 -> MASTER/4
  WD_RESET_In/1 -> Mux9/1
  COILOUTF_MASK/1 -> COILOUTF/6
  COILOUTF_CTRL/1 -> COILOUTF/5
  TEST/1(LONG_Out) -> ADD/4(TEST_L_In)
  TEST/2(PITCH_Out) -> ADD/5(TEST_P_In)
  TEST/3(YAW_Out) -> ADD/6(TEST_Y_In)
  LOCK/3 -> ADDASC/1(ISC_P_In)
  OL_TILT_SEG1/1 -> OPLEV/1(In1)
  OL_TILT_SEG2/1 -> OPLEV/2(In2)
  OL_TILT_SEG4/1 -> OPLEV/4(In4)
  OL_LEN_SEG1/1 -> OPLEV/5(In5)
  OL_LEN_SEG2/1 -> OPLEV/6(In6)
  OL_LEN_SEG3/1 -> OPLEV/7(In7)
  OL_LEN_SEG4/1 -> OPLEV/8(In8)
  OL_TILT_SEG3/1 -> OPLEV/3(In3)
  [OL_L] -> DAMP/1
  DAMP/4 -> [DAMPSTATE]
  DAMP/1 -> ADD/7(DAMP_L_In)
  [SUM_T] -> WD/1(OL_T_In)
  OPLEV/4(SUM_T) -> [SUM_T]
  OPLEV/5(SUM_L) -> [SUM_L]
  [SUM_L] -> WD/2(OL_L_In)
  [OL_L] -> OL_L_Out/1
  OPLEV/1(OL_L) -> [OL_L]
  OPLEV/2(OL_P) -> [OL_P]
  OPLEV/3(OL_Y) -> [OL_Y]
  DAMP/2 -> ADD/8(DAMP_P_In)
  DAMP/3 -> ADD/9(DAMP_Y_In)
  [OL_P] -> DAMP/2
  [OL_Y] -> DAMP/3
  ISCINF/1 -> [ISC_L], LOCK/1
  ISCINF/2 -> [ISC_P], LOCK/2
  ISCINF/3 -> [ISC_Y], LOCK/3
  [ISC_Y] -> ISC_Y_Out/1
  [ISC_P] -> ISC_P_Out/1
  [ISC_L] -> ISC_L_Out/1

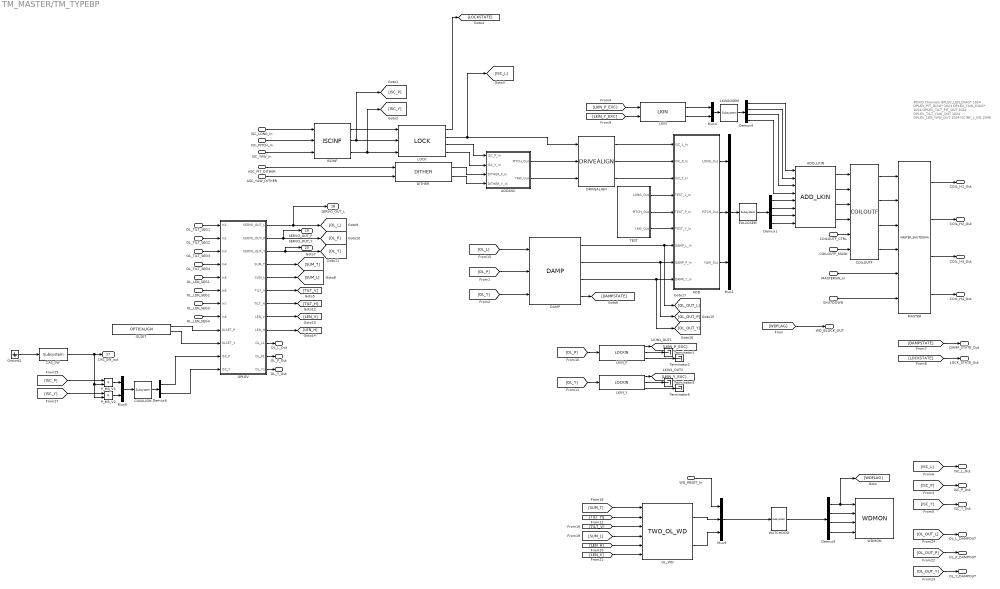
== system TM_MASTER/TM_TYPEBP ==
  note: #DAQ Channels
      | OPLEV_LEN_DIAG* 1024
      | OPLEV_PIT_DIAG* 1024
      | OPLEV_YAW_DIAG* 1024
      | OPLEV_TILT_PIT_OUT 1024
      | OPLEV_TILT_YAW_OUT 1024
      | OPLEV_LEN_YAW_OUT 1024
      | ISCINF_L_IN1 2048
  ISC_LONG_In : Inport
  ISC_PITCH_In : Inport  Port=2
  ISC_YAW_In : Inport  Port=3
  COILOUTF_CTRL : Inport  Port=4
  COILOUTF_MASK : Inport  Port=5
  OL_TILT_SEG1 : Inport  Port=6
  OL_TILT_SEG2 : Inport  Port=7
  OL_TILT_SEG3 : Inport  Port=8
  OL_TILT_SEG4 : Inport  Port=9
  OL_LEN_SEG1 : Inport  Port=10
  OL_LEN_SEG2 : Inport  Port=11
  OL_LEN_SEG3 : Inport  Port=12
  OL_LEN_SEG4 : Inport  Port=13
  MASTERSW_In : Inport  Port=14
  WD_RESET_In : Inport  Port=15
  ASC_PIT_DITHER : Inport  Port=16
  ASC_YAW_DITHER : Inport  Port=17
  SHUTDOWN : Inport  Port=18
  ADD : Subsystem
  ADDASC : Subsystem
  ADD_LKIN : VIS_LIB/ADD_LKIN
  CASALIGN : cdsMuxMatrix/Subsystem  Tag=cdsMuxMatrix  Description=Any size matrix. Inputs and outputs must be connected using Mux and Demux parts.
      settings: AttributesFormatString=%<Tag>
  CAS_SW : cdsEpicsBinIn/Subsystem  Tag=cdsEpicsBinIn  Description=|
      | Purpose:                                                                            
      | Create an EPICS binary (0 or 1) input channel to the FE realtime controls.          
      |                                                                                     
      | Operation:                                                                          
      | Outputs value from an EPICS ai record. Value is binary input (bi Epics record type).
      |                                                                                     
      | Usage:                                                                              
      | Name the part with the desired EPICS channel name.
      settings: AttributesFormatString=%<Tag>
  COILOUTF : FOUROSEM_COILOUTF_MASTER/COILOUTF
  DAMP : VIS_LIB/DAMP
  DITHER : VIS_LIB/DITHER
  DRIVEALIGN : VIS_LIB/DRIVEALIGN
  Demux1 : Demux
  Demux4 : Demux
  Demux6 : Demux  Outputs=2
  Demux9 : Demux
  EUL2OSEM : cdsMuxMatrix/Subsystem  Tag=cdsMuxMatrix  Description=Any size matrix. Inputs and outputs must be connected using Mux and Demux parts.
      settings: AttributesFormatString=%<Tag>
  Ground1 : Ground
  ISCINF : VIS_LIB/ISCINF
  LKIN : VIS_LIB/LKIN
  LKIN2OSEM : cdsMuxMatrix/Subsystem  Tag=cdsMuxMatrix  Description=Any size matrix. Inputs and outputs must be connected using Mux and Demux parts.
      settings: AttributesFormatString=%<Tag>
  LKIN_P : lockin/LOCKIN  Description=ADL=LOCKIN.adl
      settings: AttributesFormatString=%<Tag>
  LKIN_Y : lockin/LOCKIN  Description=ADL=LOCKIN.adl
      settings: AttributesFormatString=%<Tag>
  LOCK : VIS_LIB/LOCK
  MASTER : VIS_LIB/MASTER_SHUTDOWN
  Mux1 : Mux  Inputs=3
  Mux4 : Mux  Inputs=2
  Mux6 : Mux  Inputs=2
  Mux9 : Mux  Inputs=3
  OLSET : SIXOSEM_F_STAGE_MASTER/SIXOSEM_F_STAGE_TYPEBP_MASTER/OPTICALIGN
  OL_WD : OPLEV_MASTER/TWO_OL_WD
  OPLEV : Subsystem
  P_MS_V1 : Product  RndMeth=Zero
  P_MS_V2 : Product  RndMeth=Zero
  TEST : Subsystem
  Terminator{1..2,5..6} (4 alike) : Terminator
  WATCHDOG : cdsFunctionCall/Subsystem  Tag=cdsFunctionCall  Description=inline OPLEVWATCHDOG /opt/rtcds/userapps/release/vis/common/src/WATCHDOG.c
      settings: AttributesFormatString=%<Tag>\n%<Description>
  WDMON : VIS_LIB/WDMON
  COIL_H1_Out : Outport
  COIL_H2_Out : Outport  Port=2
  COIL_H3_Out : Outport  Port=3
  COIL_H4_Out : Outport  Port=4
  WD_BLOCK_OUT : Outport  Port=5
  DAMP_STATE_Out : Outport  Port=6
  LOCK_STATE_Out : Outport  Port=7
  OL_L_Out : Outport  Port=8
  OL_P_Out : Outport  Port=9
  OL_Y_Out : Outport  Port=10
  ISC_L_Out : Outport  Port=11
  ISC_P_Out : Outport  Port=12
  ISC_Y_Out : Outport  Port=13
  OL_L_DAMPOUT : Outport  Port=14
  OL_P_DAMPOUT : Outport  Port=15
  OL_Y_DAMPOUT : Outport  Port=16
  CAS_SW_out : Outport  Port=17
  SERVO_OUT_L : Outport  Port=18
  SERVO_OUT_P : Outport  Port=19
  SERVO_OUT_Y : Outport  Port=20
  wires:
  ISC_PITCH_In/1 -> ISCINF/2
  ISC_LONG_In/1 -> ISCINF/1
  ISC_YAW_In/1 -> ISCINF/3
  OL_WD/1 -> Mux9/2
  [LKIN_Y_EXC] -> LKIN/2
  [LKIN_P_EXC] -> LKIN/1
  LKIN_Y/3 -> Terminator6/1
  LKIN_Y/2 -> Terminator5/1
  [OL_Y] -> LKIN_Y/1
  LKIN_Y/1 -> [LKIN_Y_EXC]
  LKIN_P/1 -> [LKIN_P_EXC]
  LKIN_P/3 -> Terminator2/1
  LKIN_P/2 -> Terminator1/1
  [OL_P] -> LKIN_P/1
  LOCK/1 -> [LOCKSTATE]
  [LOCKSTATE] -> LOCK_STATE_Out/1
  [DAMPSTATE] -> DAMP_STATE_Out/1
  MASTERSW_In/1 -> MASTER/5
  ADD_LKIN/4 -> COILOUTF/4
  ADD_LKIN/3 -> COILOUTF/3
  ADD_LKIN/2 -> COILOUTF/2
  ADD_LKIN/1 -> COILOUTF/1
  Demux1/4 -> ADD_LKIN/8
  Demux1/3 -> ADD_LKIN/7
  Demux1/2 -> ADD_LKIN/6
  Demux1/1 -> ADD_LKIN/5
  Demux4/4 -> ADD_LKIN/4
  Demux4/3 -> ADD_LKIN/3
  Demux4/2 -> ADD_LKIN/2
  LKIN/2 -> Mux4/2
  LKIN/1 -> Mux4/1
  Demux4/1 -> ADD_LKIN/1
  LKIN2OSEM/1 -> Demux4/1
  Mux4/1 -> LKIN2OSEM/1
  MASTER/4 -> COIL_H4_Out/1
  MASTER/3 -> COIL_H3_Out/1
  MASTER/2 -> COIL_H2_Out/1
  MASTER/1 -> COIL_H1_Out/1
  DRIVEALIGN/3 -> ADD/3(ISC_Y_In)
  DRIVEALIGN/2 -> ADD/2(ISC_P_In)
  DRIVEALIGN/1 -> ADD/1(ISC_L_In)
  ADDASC/2(YAW_Out) -> DRIVEALIGN/3
  ADDASC/1(PITCH_Out) -> DRIVEALIGN/2
  LOCK/2 -> [ISC_L], DRIVEALIGN/1
  ADD/1(LONG_Out) -> Mux1/1
  ADD/2(PITCH_Out) -> Mux1/2
  ADD/3(YAW_Out) -> Mux1/3
  DITHER/2 -> ADDASC/4(DITHER_Y_In)
  DITHER/1 -> ADDASC/3(DITHER_P_In)
  LOCK/4 -> ADDASC/2(ISC_Y_In)
  ASC_YAW_DITHER/1 -> DITHER/2
  ASC_PIT_DITHER/1 -> DITHER/1
  Mux1/1 -> EUL2OSEM/1
  EUL2OSEM/1 -> Demux1/1
  Demux9/1 -> [WDFLAG], WDMON/1
  Demux9/2 -> WDMON/2
  Demux9/3 -> WDMON/3
  Demux9/4 -> WDMON/4
  WATCHDOG/1 -> Demux9/1
  Mux9/1 -> WATCHDOG/1
  [WDFLAG] -> WD_BLOCK_OUT/1
  COILOUTF/1 -> MASTER/1
  COILOUTF/2 -> MASTER/2
  COILOUTF/3 -> MASTER/3
  COILOUTF/4 -> MASTER/4
  WD_RESET_In/1 -> Mux9/1
  COILOUTF_MASK/1 -> COILOUTF/6
  COILOUTF_CTRL/1 -> COILOUTF/5
  TEST/1(LONG_Out) -> ADD/4(TEST_L_In)
  TEST/2(PITCH_Out) -> ADD/5(TEST_P_In)
  TEST/3(YAW_Out) -> ADD/6(TEST_Y_In)
  LOCK/3 -> ADDASC/1(ISC_P_In)
  OL_TILT_SEG1/1 -> OPLEV/1(In1)
  OL_TILT_SEG2/1 -> OPLEV/2(In2)
  OL_TILT_SEG4/1 -> OPLEV/4(In4)
  OL_LEN_SEG1/1 -> OPLEV/5(In5)
  OL_LEN_SEG2/1 -> OPLEV/6(In6)
  OL_LEN_SEG3/1 -> OPLEV/7(In7)
  OL_LEN_SEG4/1 -> OPLEV/8(In8)
  OL_TILT_SEG3/1 -> OPLEV/3(In3)
  [OL_L] -> DAMP/1
  DAMP/4 -> [DAMPSTATE]
  DAMP/1 -> [OL_OUT_L], ADD/7(DAMP_L_In)
  [SUM_T] -> OL_WD/1
  OPLEV/4(SUM_T) -> [SUM_T]
  OPLEV/5(SUM_L) -> [SUM_L]
  [SUM_L] -> OL_WD/4
  DAMP/2 -> [OL_OUT_P], ADD/8(DAMP_P_In)
  DAMP/3 -> [OL_OUT_Y], ADD/9(DAMP_Y_In)
  [OL_P] -> DAMP/2
  [OL_Y] -> DAMP/3
  ISCINF/1 -> LOCK/1
  ISCINF/2 -> [ISC_P], LOCK/2
  ISCINF/3 -> [ISC_Y], LOCK/3
  [ISC_Y] -> ISC_Y_Out/1
  [ISC_P] -> ISC_P_Out/1
  [ISC_L] -> ISC_L_Out/1
  SHUTDOWN/1 -> MASTER/6
  OL_WD/2 -> Mux9/3
  OPLEV/6(TILT_V) -> [TILT_V]
  OPLEV/7(TILT_H) -> [TILT_H]
  OPLEV/8(LEN_V) -> [LEN_V]
  OPLEV/9(LEN_H) -> [LEN_H]
  [TILT_H] -> OL_WD/2
  [TILT_V] -> OL_WD/3
  [LEN_H] -> OL_WD/5
  [LEN_V] -> OL_WD/6
  [OL_OUT_Y] -> OL_Y_DAMPOUT/1
  [OL_OUT_P] -> OL_P_DAMPOUT/1
  [OL_OUT_L] -> OL_L_DAMPOUT/1
  CASALIGN/1 -> Demux6/1
  Mux6/1 -> CASALIGN/1
  P_MS_V2/1 -> Mux6/2
  P_MS_V1/1 -> Mux6/1
  CAS_SW/1 -> CAS_SW_out/1, P_MS_V2/2, P_MS_V1/2
  [ISC_P] -> P_MS_V1/1
  [ISC_Y] -> P_MS_V2/1
  Ground1/1 -> CAS_SW/1
  OLSET/2 -> OPLEV/10(OLSET_Y)
  OLSET/1 -> OPLEV/9(OLSET_P)
  Demux6/1 -> OPLEV/11(ISC_P)
  Demux6/2 -> OPLEV/12(ISC_Y)
  OPLEV/10(OL_L1) -> OL_L_Out/1
  OPLEV/11(OL_P1) -> OL_P_Out/1
  OPLEV/12(OL_Y1) -> OL_Y_Out/1
  OPLEV/1(SERVO_OUT_L) -> SERVO_OUT_L/1, [OL_L]
  OPLEV/2(SERVO_OUT_P) -> SERVO_OUT_P/1, [OL_P]
  OPLEV/3(SERVO_OUT_Y) -> SERVO_OUT_Y/1, [OL_Y]
